simulink model "new"  (Simulink 7.7)
settings: Solver=ode45  StartTime=0.0  StopTime=10  RelTol=1e-3
PreLoadFcn:
  | EbNo = 16; Errors = 188; Bits = 1e8; M = 256; N = 64; Ts = (1/22050); constellation; InnerInterleaverBitTable
undefined symbols (not defined in the file or in its folder): rsgenpoly
libraries: simulink x2, commblkintrlv2 x2, commblkcod2 x1, dspsrcs4 x1, vipsrcs x1, commcnvintrlv2 x1, commcnvcod2 x1, commutil2 x1, dspxfrm3 x1, dspsigops x1, commdigbbndam3 x1, commsdrhw_v2 x1
settings Model: Creator=katsikas  LastModifiedBy=katsikas
settings SimEventsCC: propDiagAttribOutput=1  propDiagFcnCallOutput=1  propDiagStatOutput=0

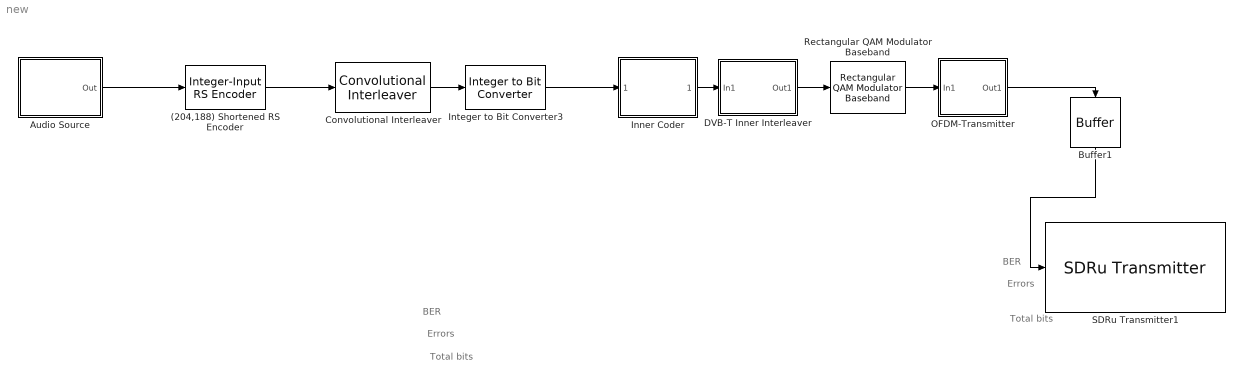
== system new ==
  note: BER
  note: Total bits
  note: Errors
  note: BER
  note: Total bits
  note: Errors
  (204,188) Shortened RS Encoder : commblkcod2/Integer-Input RS Encoder  n=204  k=188  specPrimPoly=off  prPoly=[1 0 1 1]  specGenPoly=off  genPoly=rsgenpoly(7,3)  specPuncture=off  punctVec=[ones(2,1); zeros(2,1)]
  Audio Source : Subsystem
  Buffer1 : Buffer  N=2048  TreatMby1Signals=One channel
  Convolutional Interleaver : commcnvintrlv2/Convolutional Interleaver  SystemSampleTime=-1  N=12  B=17  ic=0
  DVB-T Inner Interleaver : Subsystem  mask(DVB-T Inner Interleaver){}
      mask init:
      | fullILVec = [(1:126) ...
      |  (rem([0:125]+63,126) +1 + 126     ) ...
      |  (rem([0:125]+105,126)+1 + (2*126) ) ...
      |  (rem([0:125]+42,126) +1 + (3*126) ) ...
      |  (rem([0:125]+21,126) +1 + (4*126) ) ...
      |  (rem([0:125]+84,126) +1 + (5*126) )];
      mask Display: disp('DVB-T\nInner\nInterleaver')
  Inner Coder : Subsystem
      mask Display: disp('Rate 3/4\nPunctured\nConvolutional\nCode');
  Integer to Bit Converter3 : commutil2/Integer to Bit Converter  nbits=log2(M)  signedInputValues=Unsigned  bitOrder=MSB first  outDtype=boolean
  OFDM-Transmitter : Subsystem
  Rectangular QAM Modulator Baseband : commdigbbndam3/Rectangular QAM Modulator Baseband  M=N  InType=Bit  Enc=User-defined  Mapping=map_constellation  PowType=Average Power  MinDist=2  AvgPow=1  PeakPow=1  Ph=0  outDtype=double  outWordLen=16  outUDDataType=sfix(16)  outFracLenMode=Best precision  outFracLen=15
  SDRu Transmitter1 : commsdrhw_v2/SDRu Transmitter  SystemSampleTime=-1  rxtx=tx  USRP2_IP='192.168.10.2'  centerFrequency=794000000  centerFrequencySrc=Dialog  loOffset=0  loOffsetSrc=Dialog  gain=30  gainSrc=Dialog  decimInterp=512  decimInterpSrc=Dialog  USRP2_IP_NUM=[49 57 50 46 49 54 56 46 49 48 46 50]  frameLength=362  outputDatatype=double  overrunUnderrunPort=off  sampleTime=1  dboardInfo=|  HOST_DATA_PORT=30000  HOST_CONTROL_PORT=30001  USRP2_DATA_PORT=32769  USRP2_CONTROL_PORT=32768
      | dbid: 0
      |           dbName: 'no db found'
      |          freqMin: 0
      |          freqMax: 0
      |          gainMin: 0
      |          gainMax: 0
      |     gainStepSize: 0
  wires:
  Rectangular QAM Modulator Baseband/1 -> OFDM-Transmitter/1(In1)
  Convolutional Interleaver/1 -> Integer to Bit Converter3/1
  (204,188) Shortened RS Encoder/1 -> Convolutional Interleaver/1
  Integer to Bit Converter3/1 -> Inner Coder/1(Uncoded symbols)
  Inner Coder/1(Coded bits) -> DVB-T Inner Interleaver/1(In1)
  DVB-T Inner Interleaver/1(Out1) -> Rectangular QAM Modulator Baseband/1
  Audio Source/1(Out) -> (204,188) Shortened RS Encoder/1
  Buffer1/1 -> SDRu Transmitter1/1
  OFDM-Transmitter/1(Out1) -> Buffer1/1

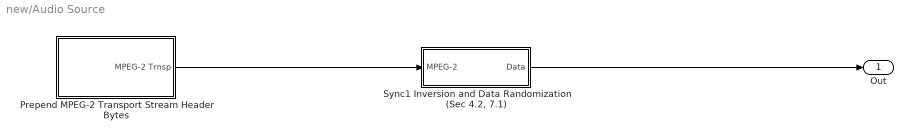
== system new/Audio Source ==
  Prepend MPEG-2 Transport Stream Header Bytes : Subsystem
      mask Display: disp(sprintf('Prepend MPEG-2\nTransportStream\nHeader Bytes'))
  "Sync1 Inversion and Data Randomization (Sec 4.2, 7.1)" : Subsystem
  Out : Outport
  wires:
  Prepend MPEG-2 Transport Stream Header Bytes/1(MPEG-2 Trnsp) -> "Sync1 Inversion and Data Randomization (Sec 4.2, 7.1)"/1(MPEG-2)
  "Sync1 Inversion and Data Randomization (Sec 4.2, 7.1)"/1(Data) -> Out/1

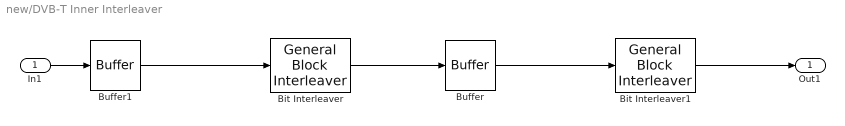
== system new/DVB-T Inner Interleaver ==
  In1 : Inport
  Bit Interleaver : commblkintrlv2/General Block Interleaver  elements=BitInterleaverTable
  Bit Interleaver1 : commblkintrlv2/General Block Interleaver  elements=SymbolInterleaverTable
  Buffer : Buffer  N=9072  TreatMby1Signals=One channel
  Buffer1 : Buffer  N=756  TreatMby1Signals=One channel
  Out1 : Outport
  wires:
  In1/1 -> Buffer1/1
  Buffer/1 -> Bit Interleaver1/1
  Buffer1/1 -> Bit Interleaver/1
  Bit Interleaver/1 -> Buffer/1
  Bit Interleaver1/1 -> Out1/1

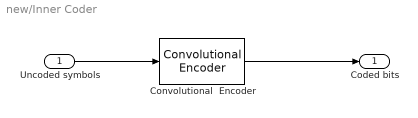
== system new/Inner Coder ==
  Uncoded symbols : Inport
  Convolutional  Encoder : commcnvcod2/Convolutional Encoder  trellis=poly2trellis(7, [171 133])  opMode=Continuous  DelayedResetAction=off  hasIniStPort=off  hasFinStPort=off  usePuncVector=on  punctureVector=[1 1 0 1 1 0]'  reset=Unused parameter value
  Coded bits : Outport
  wires:
  Convolutional  Encoder/1 -> Coded bits/1
  Uncoded symbols/1 -> Convolutional  Encoder/1

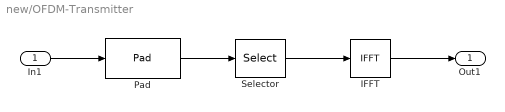
== system new/OFDM-Transmitter ==
  In1 : Inport
  IFFT : dspxfrm3/IFFT  CompMethod=Table lookup  TableOpt=NEW  TableOptActive=Speed  BitRevOrder=off  cs_in=off  SkipNorm=on  InheritFFTLength=on  FFTLength=64  mode=Complex  outSamplingMode=Frame based  RowConvenienceOn=on  firstCoeffDataTypeStr=Inherit: Same word length as input  firstCoeffLastDataTypeStr=Inherit: Same word length as input  outputMin=[]  outputMax=[]  roundingMode=Floor  overflowMode=off
  Pad : dspsigops/Pad  padAlong=Columns  dimsToPad=1  valSrc=Specify via dialog  padVal=0  spec=Output size  padNumOutRowsSpecMethod=User-specified  numOutRows=2048  padNumOutColsSpecMethod=User-specified  numOutCols=1  isVarDimsMode=off  padBeginning=0  padEnd=0  outSizeMode=User-specified  outSize=1  padSigAt=End  trunc_flag=None  roundingMode=Floor  overflowMode=off  truncOrWrapMode=Truncate  wrap_flag=None
  Selector : Selector  NumberOfDimensions=2  InputPortWidth=3  IndexOptions=Index vector (dialog),Select all  Indices=[1:756 1513:2048 757:1512],1  OutputSizes=1,1
  Out1 : Outport
  wires:
  Pad/1 -> Selector/1
  Selector/1 -> IFFT/1
  IFFT/1 -> Out1/1
  In1/1 -> Pad/1

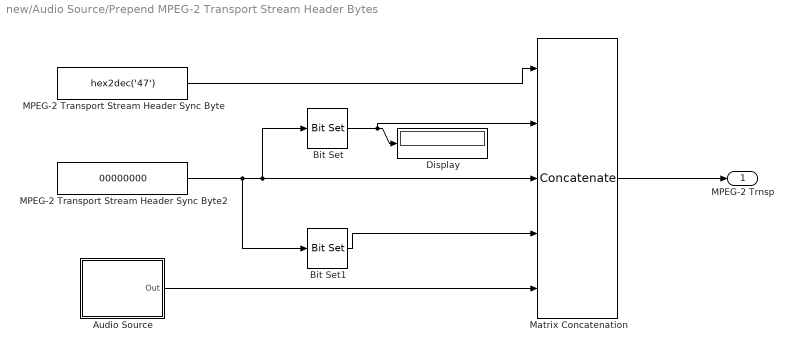
== system new/Audio Source/Prepend MPEG-2 Transport Stream Header Bytes ==
  Audio Source : Subsystem
  Bit Set : simulink/Logic and Bit Operations/Bit Set  SystemSampleTime=-1  iBit=3
  Bit Set1 : simulink/Logic and Bit Operations/Bit Set  SystemSampleTime=-1  iBit=4
  Display : Display
  MPEG-2 Transport Stream Header Sync Byte : Constant  Value=hex2dec('47')  VectorParams1D=off  OutDataTypeStr=uint8  FramePeriod=(8*188)/24e6
      settings: SamplingMode=Frame based
  MPEG-2 Transport Stream Header Sync Byte2 : Constant  Value=00000000  VectorParams1D=off  OutDataTypeStr=uint8  FramePeriod=(8*188)/24e6
      settings: SamplingMode=Frame based
  Matrix Concatenation : Concatenate  NumInputs=5  Mode=Multidimensional array
  MPEG-2 Trnsp : Outport
  wires:
  MPEG-2 Transport Stream Header Sync Byte/1 -> Matrix Concatenation/1
  Matrix Concatenation/1 -> MPEG-2 Trnsp/1
  Audio Source/1(Out) -> Matrix Concatenation/5
  MPEG-2 Transport Stream Header Sync Byte2/1 -> Bit Set1/1, Matrix Concatenation/3, Bit Set/1
  Bit Set1/1 -> Matrix Concatenation/4
  Bit Set/1 -> Display/1, Matrix Concatenation/2

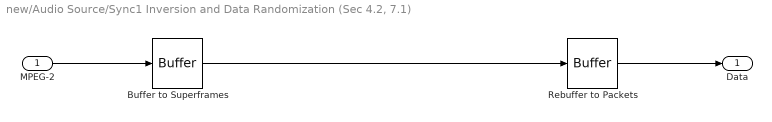
== system new/Audio Source/Sync1 Inversion and Data Randomization (Sec 4.2, 7.1) ==
  MPEG-2 : Inport
  Buffer to Superframes : Buffer  N=1504  TreatMby1Signals=One channel
  Rebuffer to Packets : Buffer  N=188  TreatMby1Signals=One channel
  Data : Outport
  wires:
  MPEG-2/1 -> Buffer to Superframes/1
  Rebuffer to Packets/1 -> Data/1
  Buffer to Superframes/1 -> Rebuffer to Packets/1

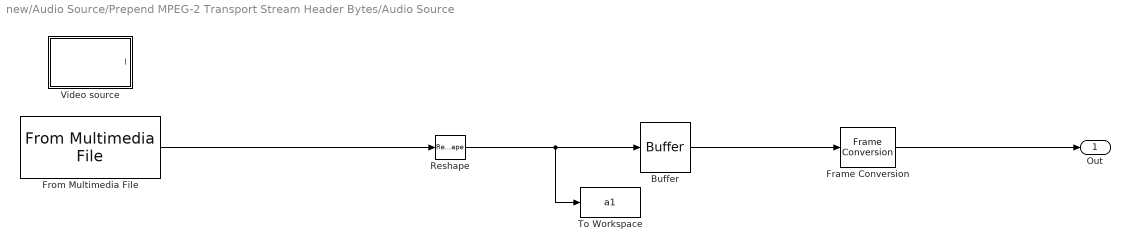
== system new/Audio Source/Prepend MPEG-2 Transport Stream Header Bytes/Audio Source ==
  Buffer : Buffer  N=184  TreatMby1Signals=One channel
  Frame Conversion : FrameConversion
  From Multimedia File : dspsrcs4/From Multimedia File  inputFilename=vipmen.avi  loop=on  numPlays=inf  outputStreams=Video only  videoDataType=uint8  audioDataType=int16  inheritSampleTime=off  userDefinedSampleTime=(8*188/24e6) / (8 * 184)  noAudioOutput=off  isIntensityVideo=off  fourcc=RGB  colorVideoFormat=One multidimensional signal  outputEOF=off  dataOrg=Column-major  audioFrameSize=1024  computeAudioFrameSize=off
  Reshape : Reshape  OutputDimensionality=Column vector (2-D)  OutputDimensions=[160,120]
  To Workspace : ToWorkspace  VariableName=a1  SampleTime=-1  SaveFormat=Array
  Video source : Subsystem
  Out : Outport
  wires:
  Reshape/1 -> Buffer/1, To Workspace/1
  Buffer/1 -> Frame Conversion/1
  Frame Conversion/1 -> Out/1
  From Multimedia File/1 -> Reshape/1

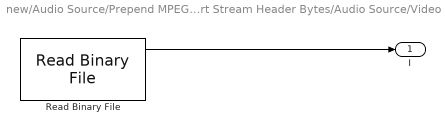
== system new/Audio Source/Prepend MPEG-2 Transport Stream Header Bytes/Audio Source/Video source ==
  Read Binary File : vipsrcs/Read Binary File  FileName=vipmen.bin  loopOrNot=on  numLoops=inf  VideoFormat=Custom  FOURCC=I420  BitStreamFormat=Planar  NumOutputs=3  ComponentOrder=[1 2 3]  Interlaced=off  LineOrdering=Top line first  Ts=(8*188/9.6e6) / (8 * 184)  Component1=Y'  Component2=Cb  Component3=Cr  Component4=Alpha  Bits1=8  Bits2=8  Bits3=8  Bits4=8  Rows1=120  Rows2=60  Rows3=60  Rows4=288  Cols1=160  Cols2=80  Cols3=80  Cols4=352  YRows=120  YCols=160  SignedOutput=off  FileEndian=Little endian  OutputEOF=off
  I : Outport
  wires:
  Read Binary File/1 -> I/1
